simulink model "Model14DOF"  (R2021b)
settings: Solver=ode23tb  StartTime=0.0  StopTime=15  RelTol=1e-3
values from neighbouring files (symbols this model uses):
  InitialLatPosition = 0    [Init_Parameters.m]
  numWheels = 4    [Init_Parameters.m]    (also in VehicleParameters.m)
  TrackWidth = VEH.TrackWidth    [Init_Parameters.m]
  VEH = data.VEH    [Init_Parameters.m]    (also in ModelWorkspace.mat = ; VehicleParameters.m)
  wheelB = VEH.FrontAxlePositionfromCG+VEH.RearAxlePositionfromCG    [Init_Parameters.m]    (also in VehicleParameters.m)
undefined symbols (not defined in the file or in its folder): degtorad
libraries: sharedtransform x5, autolibutils x3, vehdynlibsuspension x2, shared6dof x2, vehdynlibeom x1, vehdynlibtire x1, vehdynlibtirecommon x1
(part 1 of 2)
settings Model: Creator=monic  LastModifiedBy=monic

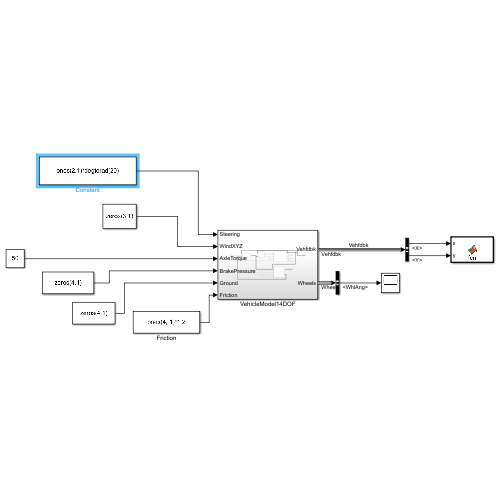
[thumbnail: Simulink's stored preview of the top-level diagram]
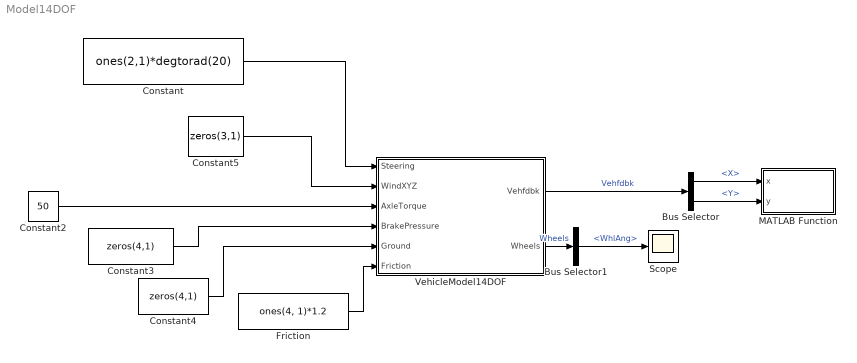
== system Model14DOF ==
  Bus Selector : BusSelector  OutputSignals=InertFrm.Cg.Disp.X,InertFrm.Cg.Disp.Y
  Bus Selector1 : BusSelector  OutputSignals=Steering.WhlAng
  Constant : Constant  Value=ones(2,1)*degtorad(20)
  Constant2 : Constant  Value=50
  Constant3 : Constant  Value=zeros(4,1)
  Constant4 : Constant  Value=zeros(4,1)
  Constant5 : Constant  Value=zeros(3,1)
  Friction : Constant  Value=ones(4, 1)*1.2
  MATLAB Function : MATLAB Function  TreatAsAtomicUnit=on
  Scope : Scope
  VehicleModel14DOF : Subsystem
  wires:
  Constant/1 -> VehicleModel14DOF/1(Steering)
  Constant5/1 -> VehicleModel14DOF/2(WindXYZ)
  Constant2/1 -> VehicleModel14DOF/3(AxleTorque)
  Constant3/1 -> VehicleModel14DOF/4(BrakePressure)
  Constant4/1 -> VehicleModel14DOF/5(Ground)
  Friction/1 -> VehicleModel14DOF/6(Friction)
  VehicleModel14DOF/2(Wheels) -> Bus Selector1/1  "Wheels"
  VehicleModel14DOF/1(Vehfdbk) -> Bus Selector/1  "Vehfdbk"
  Bus Selector/2 -> MATLAB Function/2(y)  "<Y>"
  Bus Selector/1 -> MATLAB Function/1(x)  "<X>"
  Bus Selector1/1 -> Scope/1  "<WhlAng>"

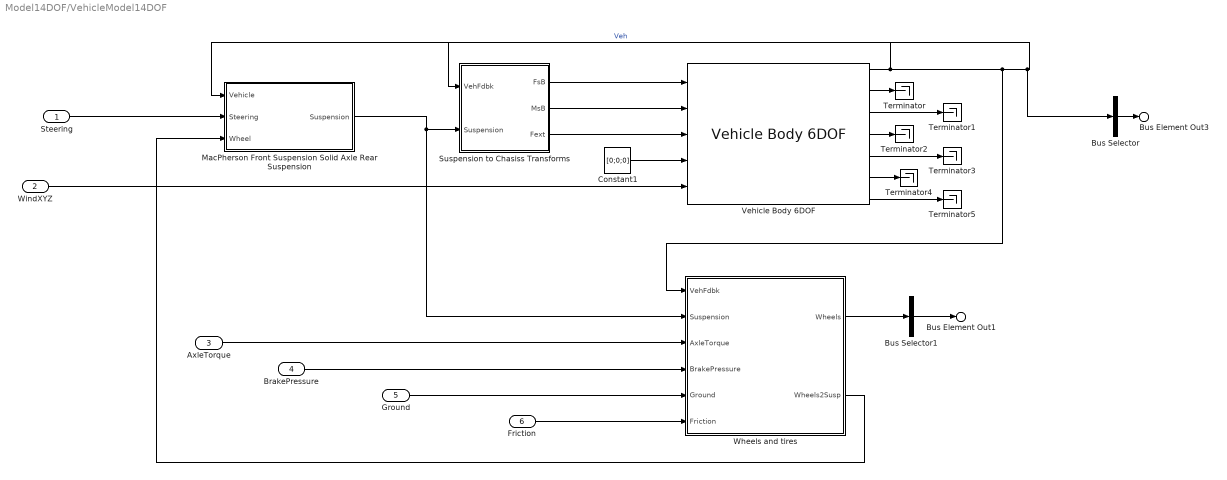
== system Model14DOF/VehicleModel14DOF ==
  Steering : Inport
  WindXYZ : Inport  Port=2
  AxleTorque : Inport  Port=3
  BrakePressure : Inport  Port=4
  Ground : Inport  Port=5
  Friction : Inport  Port=6
  Bus Selector : BusSelector  OutputSignals=InertFrm,BdyFrm  OutputAsBus=on
  Bus Selector1 : BusSelector  OutputSignals=TireFrame,Steering  OutputAsBus=on
  Constant1 : Constant  Value=[0;0;0]
  MacPherson Front Suspension Solid Axle Rear Suspension : Subsystem
  Suspension to Chasiss Transforms : Subsystem
  Terminator{,1..5} (6 alike) : Terminator
  Vehicle Body 6DOF : vehdynlibeom/Vehicle Body 6DOF  extPos=on  extVel=on  extEuler=on  extRotRate=on  htchFMode=off  htchMMode=off  m=VEH.Mass  a=VEH.FrontAxlePositionfromCG  b=VEH.RearAxlePositionfromCG  d=0  h=VEH.HeightCG  dh=1  hl=0  hh=0.1  Xe_o=[VEH.InitialLongPosition,InitialLatPosition,VEH.InitialVertPosition]  xbdot_o=[VEH.InitialLongVel,VEH.InitialLatVel,VEH.InitialVertVel]  eul_o=[VEH.InitialRollAngle,VEH.InitialPitchAngle,VEH.InitialYawAngle]  p_o=[VEH.InitialRollRate,VEH.InitialPitchRate,VEH.InitialYawRate]  Iveh=[VEH.RollMomentInertia 0 0; 0 VEH.PitchMomentInertia 0; 0 0 VEH.YawMomentInertia]  w=VEH.TrackWidth.*[1 1]  z1m=0  z1R=[-.25,.125,.15]  z1I=[1.4,-.2,.1;-.2,1.4,.1;.1,.1,2.25].*0  z2m=0  z2R=[1.4,0,.8]  z2I=[1.4,-.2,.1;-.2,1.4,.1;.1,.1,2.25].*0  z3m=0  z3R=[.75,-.5,.4]  z3I=[5,-.1,-2;-2,9,.1;-.1,.1,6].*0  z4m=0  z4R=[.75,.5,.4]  z4I=[5,-.1,-2;-2,9,.1;-.1,.1,6].*0  z5m=0  z5R=[1.25,-.5,.4]  z5I=[5,-.1,-2;-2,9,.1;-.1,.1,6].*0  z6m=0  z6R=[1.25,-.5,.4]  z6I=[5,-.1,-2;-2,9,.1;-.1,.1,6].*0  z7m=0  z7R=[2,0,.25]  z7I=[1.4,-.2,.1;-.2,1.4,.1;.1,.1,2.25].*0  Af=VEH.FrontalArea  Cd=.3  Cl=.1  Cpm=.1  beta_w=[0 0.01:0.01:0.3]  Cs=[0 0.01:0.01:0.3]  Cym=[0 1e-6:0.01:0.3]  Pabs=101325  extTamb=off  Tair=273  g=9.81  xdot_tol=.1  longOff=0  latOff=0  vertOff=0.0112  wrapAng=off  aMode=2
      settings: SourceProductBaseCode=VE
  Wheels and tires : Subsystem
  Bus Element Out3 : Outport  PortName=Vehfdbk
  Bus Element Out1 : Outport  Port=2  PortName=Wheels
  wires:
  Ground/1 -> Wheels and tires/5(Ground)
  MacPherson Front Suspension Solid Axle Rear Suspension/1(Suspension) -> Wheels and tires/2(Suspension), Suspension to Chasiss Transforms/2(Suspension)
  Vehicle Body 6DOF/3 -> Terminator1/1
  Suspension to Chasiss Transforms/3(Fext) -> Vehicle Body 6DOF/3
  Vehicle Body 6DOF/7 -> Terminator5/1
  BrakePressure/1 -> Wheels and tires/4(BrakePressure)
  AxleTorque/1 -> Wheels and tires/3(AxleTorque)
  Vehicle Body 6DOF/6 -> Terminator4/1
  Vehicle Body 6DOF/5 -> Terminator3/1
  Constant1/1 -> Vehicle Body 6DOF/4
  Wheels and tires/2(Wheels2Susp) -> MacPherson Front Suspension Solid Axle Rear Suspension/3(Wheel)
  Vehicle Body 6DOF/4 -> Terminator2/1
  Suspension to Chasiss Transforms/1(FsB) -> Vehicle Body 6DOF/1
  Vehicle Body 6DOF/2 -> Terminator/1
  Suspension to Chasiss Transforms/2(MsB) -> Vehicle Body 6DOF/2
  WindXYZ/1 -> Vehicle Body 6DOF/5
  Steering/1 -> MacPherson Front Suspension Solid Axle Rear Suspension/2(Steering)
  Friction/1 -> Wheels and tires/6(Friction)
  Wheels and tires/1(Wheels) -> Bus Selector1/1
  Bus Selector1/1 -> Bus Element Out1/1
  Vehicle Body 6DOF/1 -> Wheels and tires/1(VehFdbk), Bus Selector/1, MacPherson Front Suspension Solid Axle Rear Suspension/1(Vehicle), Suspension to Chasiss Transforms/1(VehFdbk)  "Veh"
  Bus Selector/1 -> Bus Element Out3/1

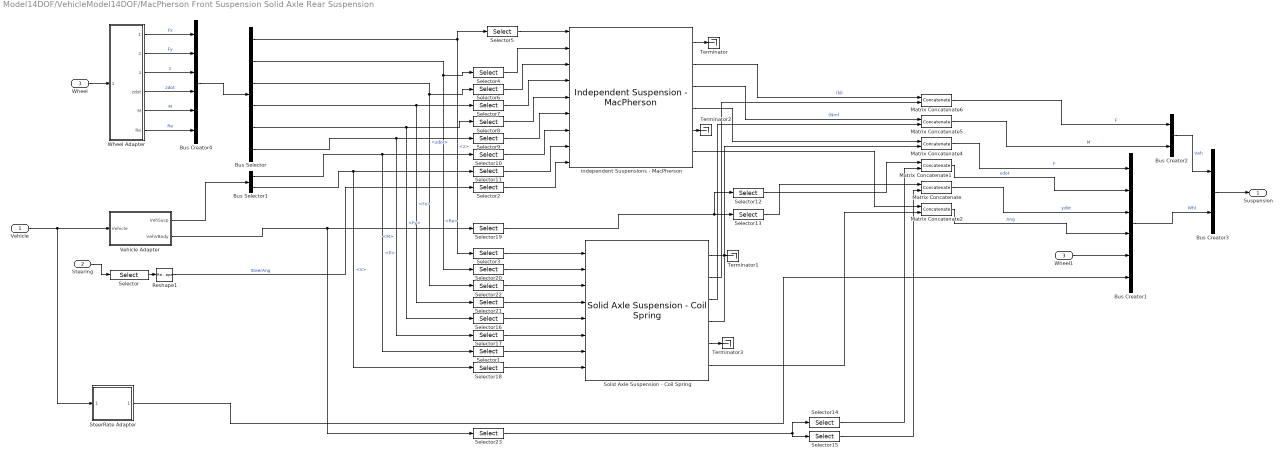
== system Model14DOF/VehicleModel14DOF/MacPherson Front Suspension Solid Axle Rear Suspension ==
  Vehicle : Inport
  Steering : Inport  Port=2
  Wheel : Inport  Port=3
  Bus Creator1 : BusCreator  Inputs=6
  Bus Creator2 : BusCreator  Inputs=2
  Bus Creator3 : BusCreator  Inputs=2
  Bus Creator4 : BusCreator  Inputs=6
  Bus Selector : BusSelector  OutputSignals=z,Re,zdot,Fx,Fy,M
  Bus Selector1 : BusSelector  OutputSignals=P,V
  Matrix Concatenate{,1..2,4..6} (6 alike) : Concatenate  Mode=Multidimensional array  ConcatenateDimension=2
  Reshape1 : Reshape  OutputDimensionality=Row vector (2-D)
  Selector{,2,4..8} (7 alike) : Selector  IndexOptions=Index vector (dialog)  Indices=[1 2]  OutputSizes=1
  Selector{1,17..18,23} (4 alike) : Selector  NumberOfDimensions=2  IndexOptions=Select all,Index vector (dialog)  Indices=[1 2],[3 4]  OutputSizes=1,1
  Selector{9..11,19} (4 alike) : Selector  NumberOfDimensions=2  IndexOptions=Select all,Index vector (dialog)  Indices=[1 2],[1 2]  OutputSizes=1,1
  Selector12 : Selector  NumberOfDimensions=2  InputPortWidth=3  IndexOptions=Index vector (dialog),Select all  Indices=1,1  OutputSizes=1,1
  Selector13 : Selector  NumberOfDimensions=2  InputPortWidth=3  IndexOptions=Index vector (dialog),Select all  Indices=2,1  OutputSizes=1,1
  Selector14 : Selector  NumberOfDimensions=2  InputPortWidth=3  IndexOptions=Index vector (dialog),Select all  Indices=1,1  OutputSizes=1,1
  Selector15 : Selector  NumberOfDimensions=2  InputPortWidth=3  IndexOptions=Index vector (dialog),Select all  Indices=2,1  OutputSizes=1,1
  Selector{3,16,20..22} (5 alike) : Selector  IndexOptions=Index vector (dialog)  Indices=[3 4]  OutputSizes=1
  Solid Axle Suspension - Coil Spring : vehdynlibsuspension/Solid Axle Suspension - Coil Spring  NumAxl=1  NumTracksByAxl=2  StrgEnByAxl=0  TrackNumVec="[1  2]"  AxleNumVec="[1  1]"  SuspTypesByAxle=[1]  SuspImage=suspsacoil.png  AxlIxx=AxlIxx  AxlM=AxlM  TrackCoords=[0 0;VEH.TrackWidth*[-1 1]/2;0 0]  SuspCoords=[0 0;VEH.TrackWidth*[-1 1]/2;0 0]  KzWhlAxl=KzWhlAxl  F0zWhlAxl=F0zWhlAxl  CzWhlAxl=CzWhlAxl  IdealSuspEn=on  IdealSuspAxles=[1]  Kz=Kz  F0z=F0zCS  Cz=Cz  Hmax=Hmax  Toe=0.  RollStrgSlp=0.  ToeStrgSlp=0  Caster=0.  CasterHslp=0.  CasterStrgSlp=0.01  Camber=0.  CamberHslp=0.  CamberStrgSlp=0.01  StrgHgtSlp=0.1432  MappedSuspEn=off  MappedSuspAxles="[1  2]"  f_susp_axl_bp=[1 2]  f_susp_dz_bp=[-0.15 -0.14 -0.13 -0.12 -0.11 -0.10 -0.09 -0.08 -0.07 -0.06 -0.05 -0.04 -0.03 -0.02 -0.01 0.00 0.01 0.02 0.03 0.04 0.05 0.06 0.07 0.08 0.09 0.10 0.11 0.12 0.13 0.14 0.15]  f_susp_dzdot_bp=[-0.15 -0.14 -0.13 -0.12 -0.11 -0.10 -0.09 -0.08 -0.07 -0.06 -0.05 -0.04 -0.03 -0.02 -0.01 0.00 0.01 0.02 0.03 0.04 0.05 0.06 0.07 0.08 0.09 0.10 0.11 0.12 0.13 0.14 0.15]  f_susp_fmz=zeros(31,31,61,2,4)  f_susp_geom=zeros(31,61,2,3)  f_susp_strgdelta_bp=[-30,-29,-28,-27,-26,-25,-24,-23,-22,-21,-20,-19,-18,-17,-16,-15,-14,-13,-12,-11,-10,-9,-8,-7,-6,-5,-4,-3,-2,-1,0,1,2,3,4,5,6,7,8,9,10,11,12,13,14,15,16,17,18,19,20,21,22,23,24,25,26,27,28,29,30]
      settings: SourceProductBaseCode=VE
  SteerRate Adapter : Subsystem
  Terminator{,1..3} (4 alike) : Terminator
  Vehicle Adapter : Subsystem
  Wheel Adapter : Subsystem
  Wheel1 : InportShadow  Port=3
  independent Suspensions - MacPherson : vehdynlibsuspension/Independent Suspension - MacPherson  ActiveDampEn=off  NumAxl=1  NumTracksByAxl=2  StrgEnByAxl=1  AntiSwayEnByAxl=1  TrackNumVec="[1  2]"  AxleNumVec="[1  1]"  SuspTypesByAxle=[1]  SuspImage=suspmacp.png  IdealSuspEn=on  IdealSuspAxles=[1]  Kz=Kz  F0z=F0zMP  Cz=Cz  Hmax=Hmax  f_act_susp_cz=[10000 10000;10000 10000]  f_act_susp_duty_bpt=[0 1]  f_act_susp_zdot_bpt=[-1 1]  Toe=0  RollStrgSlp=0.  ToeStrgSlp=0.  Caster=0.  CasterHslp=0.  CasterStrgSlp=0.  Camber=-0.5*pi/180*0  CamberHslp=0.  CamberStrgSlp=0.  StrgHgtSlp=0.1432  MappedSuspEn=off  MappedSuspAxles="[1  2]"  f_susp_axl_bp=[1 2]  f_susp_dz_bp=[-0.15 -0.14 -0.13 -0.12 -0.11 -0.10 -0.09 -0.08 -0.07 -0.06 -0.05 -0.04 -0.03 -0.02 -0.01 0.00 0.01 0.02 0.03 0.04 0.05 0.06 0.07 0.08 0.09 0.10 0.11 0.12 0.13 0.14 0.15]  f_susp_dzdot_bp=[-0.15 -0.14 -0.13 -0.12 -0.11 -0.10 -0.09 -0.08 -0.07 -0.06 -0.05 -0.04 -0.03 -0.02 -0.01 0.00 0.01 0.02 0.03 0.04 0.05 0.06 0.07 0.08 0.09 0.10 0.11 0.12 0.13 0.14 0.15]  f_susp_fmz=zeros(31,31,61,2,4)  f_susp_geom=zeros(31,61,2,3)  f_susp_strgdelta_bp=[-30,-29,-28,-27,-26,-25,-24,-23,-22,-21,-20,-19,-18,-17,-16,-15,-14,-13,-12,-11,-10,-9,-8,-7,-6,-5,-4,-3,-2,-1,0,1,2,3,4,5,6,7,8,9,10,11,12,13,14,15,16,17,18,19,20,21,22,23,24,25,26,27,28,29,30]  AntiSwayR=0.2  AntiSwayNtrlAng=0.5236  AntiSwayTrsK=8e+02
      settings: SourceProductBaseCode=VE
  Suspension : Outport  VectorParamsAs1DForOutWhenUnconnected=off
  wires:
  Wheel1/1 -> Bus Creator1/5
  Bus Selector/5 -> Selector16/1, Selector8/1  "<Fy>"
  Vehicle Adapter/2(VehVBody) -> Selector23/1, Selector19/1
  Matrix Concatenate1/1 -> Bus Creator1/2  "xdot"
  Selector19/1 -> Selector12/1, Selector13/1
  Selector2/1 -> independent Suspensions - MacPherson/9
  Wheel Adapter/2(WhFy) -> Bus Creator4/2  "Fy"
  Selector11/1 -> independent Suspensions - MacPherson/8
  Bus Creator4/1 -> Bus Selector/1
  Bus Selector/2 -> Selector20/1, Selector4/1  "<Re>"
  Bus Selector1/2 -> Selector18/1, Selector11/1  "<V>"
  Solid Axle Suspension - Coil Spring/3 -> Matrix Concatenate5/2
  Vehicle/1 -> SteerRate Adapter/1(Vehicle), Vehicle Adapter/1(Vehicle)
  Solid Axle Suspension - Coil Spring/6 -> Matrix Concatenate2/2
  Solid Axle Suspension - Coil Spring/1 -> Terminator1/1
  Matrix Concatenate/1 -> Bus Creator1/3  "ydot"
  independent Suspensions - MacPherson/1 -> Terminator/1
  Wheel Adapter/5(M) -> Bus Creator4/5  "M"
  Selector10/1 -> independent Suspensions - MacPherson/7
  Selector23/1 -> Selector15/1, Selector14/1
  Wheel/1 -> Wheel Adapter/1(Wheels)
  Wheel Adapter/4(zdot) -> Bus Creator4/4  "zdot"
  Selector17/1 -> Solid Axle Suspension - Coil Spring/6
  Wheel Adapter/1(WhFx) -> Bus Creator4/1  "Fx"
  Selector20/1 -> Solid Axle Suspension - Coil Spring/2
  Selector6/1 -> independent Suspensions - MacPherson/3
  Selector15/1 -> Matrix Concatenate/2
  Steering/1 -> Selector/1
  Selector18/1 -> Solid Axle Suspension - Coil Spring/8
  Selector16/1 -> Solid Axle Suspension - Coil Spring/5
  Selector7/1 -> independent Suspensions - MacPherson/4
  Matrix Concatenate4/1 -> Bus Creator1/1  "F"
  Solid Axle Suspension - Coil Spring/4 -> Matrix Concatenate4/2
  Selector8/1 -> independent Suspensions - MacPherson/5
  independent Suspensions - MacPherson/2 -> Matrix Concatenate6/1  "(N)"
  Selector5/1 -> independent Suspensions - MacPherson/1
  Selector9/1 -> independent Suspensions - MacPherson/6
  Selector21/1 -> Solid Axle Suspension - Coil Spring/4
  Bus Selector1/1 -> Selector1/1, Selector10/1  "<P>"
  Selector3/1 -> Solid Axle Suspension - Coil Spring/1
  Solid Axle Suspension - Coil Spring/5 -> Terminator3/1
  Selector/1 -> Reshape1/1
  Bus Creator2/1 -> Bus Creator3/1  "Veh"
  Wheel Adapter/3(z) -> Bus Creator4/3  "z"
  Bus Selector/3 -> Selector22/1, Selector6/1  "<zdot>"
  Wheel Adapter/6(Re) -> Bus Creator4/6  "Re"
  Selector22/1 -> Solid Axle Suspension - Coil Spring/3
  Matrix Concatenate5/1 -> Bus Creator2/2  "M"
  independent Suspensions - MacPherson/4 -> Matrix Concatenate4/1
  Selector4/1 -> independent Suspensions - MacPherson/2
  Selector1/1 -> Solid Axle Suspension - Coil Spring/7
  Bus Selector/1 -> Selector3/1, Selector5/1  "<z>"
  Bus Selector/6 -> Selector17/1, Selector9/1  "<M>"
  Matrix Concatenate6/1 -> Bus Creator2/1  "F"
  Bus Creator3/1 -> Suspension/1
  Bus Selector/4 -> Selector21/1, Selector7/1  "<Fx>"
  Reshape1/1 -> Selector2/1  "SteerAng"
  independent Suspensions - MacPherson/5 -> Terminator2/1
  Vehicle Adapter/1(VehSusp) -> Bus Selector1/1
  Bus Creator1/1 -> Bus Creator3/2  "Whl"
  independent Suspensions - MacPherson/3 -> Matrix Concatenate5/1  "(Nm)"
  Selector12/1 -> Matrix Concatenate1/1
  Matrix Concatenate2/1 -> Bus Creator1/4  "Ang"
  Solid Axle Suspension - Coil Spring/2 -> Matrix Concatenate6/2
  Selector14/1 -> Matrix Concatenate1/2
  independent Suspensions - MacPherson/6 -> Matrix Concatenate2/1
  Selector13/1 -> Matrix Concatenate/1
  SteerRate Adapter/1(AngVel) -> Bus Creator1/6

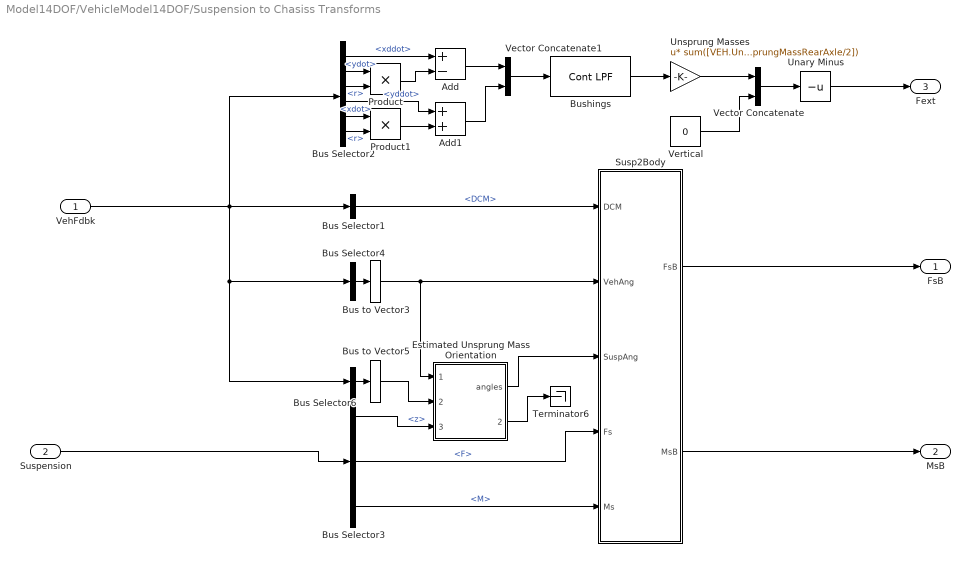
== system Model14DOF/VehicleModel14DOF/Suspension to Chasiss Transforms ==
  VehFdbk : Inport
  Suspension : Inport  Port=2
  Add : Sum  Inputs=+-
  Add1 : Sum
  Bus Selector1 : BusSelector  OutputSignals=BdyFrm.Cg.DCM
  Bus Selector2 : BusSelector  OutputSignals=BdyFrm.Cg.Acc.xddot,BdyFrm.Cg.Vel.ydot,BdyFrm.Cg.AngVel.r,BdyFrm.Cg.Acc.yddot,BdyFrm.Cg.Vel.xdot,BdyFrm.Cg.AngVel.r
  Bus Selector3 : BusSelector  OutputSignals=Whl.signal5.SuspFrame.z,Veh.F,Veh.M
  Bus Selector4 : BusSelector  OutputSignals=InertFrm.Cg.Ang.phi,InertFrm.Cg.Ang.theta,InertFrm.Cg.Ang.psi  OutputAsBus=on
  Bus Selector6 : BusSelector  OutputSignals=InertFrm.Geom.Disp.X,InertFrm.Geom.Disp.Y,InertFrm.Geom.Disp.Z  OutputAsBus=on
  Bus to Vector3 : BusToVector
  Bus to Vector5 : BusToVector
  Bushings : autolibutils/Cont LPF  wc=40*pi  aMode=2
      settings: SourceProductBaseCode=PW,DR,MT,UV,VE
  Estimated Unsprung Mass Orientation : MATLAB Function  TreatAsAtomicUnit=on
  Product : Product
  Product1 : Product
  Susp2Body : Subsystem
  Terminator6 : Terminator
  Unary Minus : UnaryMinus
  Unsprung Masses : Gain  Gain=sum([VEH.UnsprungMassFrontAxle/2 VEH.UnsprungMassFrontAxle/2 VEH.UnsprungMassRearAxle/2 VEH.UnsprungMassRearAxle/2])  Multiplication=Matrix(u*K)
  Vector Concatenate : Concatenate
  Vector Concatenate1 : Concatenate
  Vertical : Constant  Value=0
  FsB : Outport
  MsB : Outport  Port=2
  Fext : Outport  Port=3
  wires:
  Estimated Unsprung Mass Orientation/1(angles) -> Susp2Body/3(SuspAng)
  Bus Selector3/1 -> Estimated Unsprung Mass Orientation/3(Ground)  "<z>"
  Vector Concatenate1/1 -> Bushings/1
  Bus Selector2/6 -> Product1/2  "<r>"
  Product/1 -> Add/2
  Bus Selector2/3 -> Product/2  "<r>"
  Bus Selector2/5 -> Product1/1  "<xdot>"
  Vertical/1 -> Vector Concatenate/2
  Add1/1 -> Vector Concatenate1/2
  Suspension/1 -> Bus Selector3/1
  Bushings/1 -> Unsprung Masses/1
  Vector Concatenate/1 -> Unary Minus/1
  VehFdbk/1 -> Bus Selector6/1, Bus Selector4/1, Bus Selector2/1, Bus Selector1/1
  Product1/1 -> Add1/2
  Bus to Vector3/1 -> Estimated Unsprung Mass Orientation/1(angleIn), Susp2Body/2(VehAng)
  Bus to Vector5/1 -> Estimated Unsprung Mass Orientation/2(GemoXYZIn)
  Unary Minus/1 -> Fext/1
  Bus Selector2/1 -> Add/1  "<xddot>"
  Add/1 -> Vector Concatenate1/1
  Bus Selector3/3 -> Susp2Body/5(Ms)  "<M>"
  Bus Selector2/2 -> Product/1  "<ydot>"
  Unsprung Masses/1 -> Vector Concatenate/1
  Estimated Unsprung Mass Orientation/2(GeomXYZ) -> Terminator6/1
  Bus Selector2/4 -> Add1/1  "<yddot>"
  Bus Selector3/2 -> Susp2Body/4(Fs)  "<F>"
  Bus Selector1/1 -> Susp2Body/1(DCM)  "<DCM>"
  Bus Selector6/1 -> Bus to Vector5/1
  Bus Selector4/1 -> Bus to Vector3/1
  Susp2Body/1(FsB) -> FsB/1
  Susp2Body/2(MsB) -> MsB/1

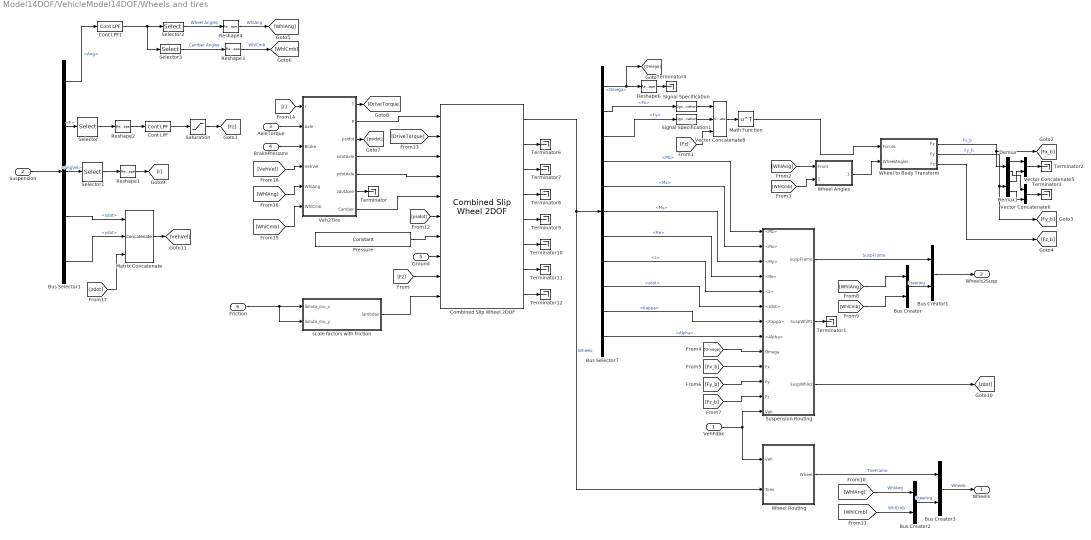
== system Model14DOF/VehicleModel14DOF/Wheels and tires ==
  VehFdbk : Inport
  Suspension : Inport  Port=2
  AxleTorque : Inport  Port=3
  BrakePressure : Inport  Port=4
  Ground : Inport  Port=5
  Friction : Inport  Port=6
  Bus Creator{,1..3} (4 alike) : BusCreator  Inputs=2
  Bus Selector1 : BusSelector  OutputSignals=Whl.Ang,Whl.F,Whl.AngVel,Whl.xdot,Whl.ydot
  Bus Selector7 : BusSelector  OutputSignals=Omega,Fx,Fy,Mz,Mx,My,Re,z,zdot,Kappa,Alpha
  Combined Slip Wheel 2DOF : vehdynlibtire/Combined Slip Wheel 2DOF  tireType=Light passenger car 205/60R15  BrakeType=Disc  plySteer=off  turnslip=off  mu_static=.3  mu_kinetic=.2  disk_abore=.05  Rm=.177  num_pads=2  drum_abore=0.0508  drum_a=0.123  drum_c=0.212  drum_r=0.15  drum_theta1=0  drum_theta2=126  brake_p_bpt=[1 11.4736842105263 21.9473684210526 32.4210526315789 42.8947368421053 53.3684210526316 63.8421052631579 74.3157894736842 84.7894736842105 95.2631578947368 105.736842105263 116.210526315789 126.684210526316 137.157894736842 147.631578947368 158.105263157895 168.578947368421 179.052631578947 189.526315789474 200]  brake_n_bpt=[0 52.6315789473684 105.263157894737 157.894736842105 210.526315789474 263.157894736842 315.789473684211 368.421052631579 421.052631578947 473.684210526316 526.315789473684 578.947368421053 631.578947368421 684.210526315789 736.842105263158 789.473684210526 842.105263157895 894.736842105263 947.368421052632 1000]  f_brake_t=[43.4900602404453 42.5056030554862 41.5350898940194 40.5780454442085 39.6340111501808 38.7025443887544 37.7832176914519 36.8756180088306 35.9793460143796 35.0940154454303 34.2192524787115 33.3546951383474 32.4999927342521 31.6548053290159 30.8188032315107 29.991666515561 29.1730845621415 28.362755623661 27.5603864089927 26.765691687993;498.991217495636 487.695866636631 476.560505099801 465.579679307235 454.748127933653 444.060772460445 433.51270824929 423.099196101319 412.81565427025 402.657650900201 392.620896861006 382.701238955775 372.894653477208 363.197240090814 353.605216024701 344.114910546964 334.722759712992 325.425301366216 316.219170376863 307.10109410434;954.492374750826 932.886130217776 911.585920305583 890.581313170261 869.862244717126 849.419000532136 829.242198807128 809.322774193808 789.651962526121 770.221286354971 751.0225412433 732.047782773203 713.289314220164 694.739674852612 676.391628817892 658.238154578366 640.272434863842 622.48784710877 604.877954344734 587.436496520688;1409.99353200602 1378.07639379892 1346.61133551136 1315.58294703329 1284.9763615006 1254.77722860383 1224.97168936497 1195.5463522863 1166.48827078199 1137.78492180974 1109.42418562559 1081.39432659063 1053.68397496312 1026.28210961441 999.178041611083 972.361398609768 945.822110014692 919.550392851325 893.536738312604 867.771898937035;1865.49468926121 1823.26665738007 1781.63675071715 1740.58458089631 1700.09047828407 1660.13545667552 1620.7011799228 1581.76993037878 1543.32457903786 1505.34855726451 1467.82583000789 1430.74087040806 1394.07863570608 1357.82454437621 1321.96445440427 1286.48464264117 1251.37178516554 1216.61293859388 1182.19552228048 1148.10730135338;2320.9958465164 2268.45692096121 2216.66216592293 2165.58621475934 2115.20459506754 2065.49368474721 2016.43067048064 1967.99350847127 1920.16088729373 1872.91219271928 1826.22747439018 1780.08741422549 1734.47329644903 1689.36697913801 1644.75086719747 1600.60788667257 1556.92146031639 1513.67548433643 1470.85430624835 1428.44270376973;2776.49700377159 2713.64718454235 2651.68758112871 2590.58784862237 2530.31871185102 2470.8519128189 2412.16016103848 2354.21708656376 2296.9971955496 2240.47582817405 2184.62911877248 2129.43395804292 2074.86795719199 2020.9094138998 1967.53727999066 1914.73113070398 1862.47113546724 1810.73803007899 1759.51309021622 1708.77810618608;3231.99816102678 3158.8374481235 3086.71299633449 3015.58948248539 2945.43282863449 2876.21014089059 2807.88965159632 2740.44066465625 2673.83350380547 2608.03946362882 2543.03076315477 2478.78050186034 2415.26261793494 2352.4518486616 2290.32369278385 2228.85437473538 2168.02081061809 2107.80057582154 2048.17187418409 1989.11350860242;3687.49931828197 3604.02771170464 3521.73841154027 3440.59111634842 3360.54694541796 3281.56836896228 3203.61914215416 3126.66424274874 3050.66981206134 2975.60309908359 2901.43240753707 2828.12704567777 2755.6572786779 2683.9942834234 2613.11010557704 2542.97761876678 2473.57048576894 2404.8631215641 2336.83065815196 2269.44891101877;4143.00047553716 4049.21797528579 3956.76382674606 3865.59275021144 3775.66106220143 3686.92659703397 3599.34863271199 3512.88782084123 3427.50612031721 3343.16673453836 3259.83405191936 3177.4735894952 3096.05193942085 3015.5367181852 2935.89651837023 2857.10086279818 2779.12016091979 2701.92566730665 2625.48944211983 2549.78431343512;4598.50163279235 4494.40823886693 4391.78924195184 4290.59438407447 4190.77517898491 4092.28482510566 3995.07812326983 3899.11139893372 3804.34242857308 3710.73036999313 3618.23569630166 3526.82013331263 3436.44660016381 3347.079152947 3258.68293116342 3171.22410682959 3084.66983607064 2998.98821304921 2914.1482260877 2830.11971585147;5054.00279004754 4939.59850244808 4826.81465715762 4715.59601793749 4605.88929576838 4497.64305317735 4390.80761382767 4285.3349770262 4181.17873682896 4078.2940054479 3976.63734068395 3876.16667713006 3776.84126090677 3678.62158770879 3581.46934395661 3485.34735086099 ...(+2764 chars)]  tireParamSet=vdynPassCar.mat  PRESMAX=1000000  PRESMIN=10000  FZMAX=10000  FZMIN=100  VXLOW=.1  KPUMAX=1.5  KPUMIN=-1.5  ALPMAX=1.5  ALPMIN=-1.5  CAMMAX=0.2  CAMMIN=-0.2  LONGVL=16.7  FxRelFreqLwrLim=200*pi  FyRelFreqLwrLim=50*pi  MyRelFreqLwrLim=100*pi  omegao=0  br=1e-3  UNLOADED_RADIUS=0.30938  NOMPRES=220000  FNOMIN=4000  WIDTH=0.20905  RIM_RADIUS=0.1914  MASS=9.4649  IYY=0.74063  GRAVITY=-9.81  zo=.015+VEH.InitialVertPosition  zdoto=0  BREFF=8.25094594147963  DREFF=0.260468730454265  FREFF=0.0735298544471851  Q_RE0=1.00866439868088  Q_V1=0.000760413786224011  Q_V2=0.0463384792019201  Q_FZ1=0  Q_FZ2=15.6870832810226  Q_FZ3=0  Q_FCX=0.138643970247602  Q_FCY=0.10843499565426  Q_FCY2=-0.465763352339538  PFZ1=0.69958166705601  VERTICAL_STIFFNESS=207885.061134007  VERTICAL_DAMPING=500  BOTTOM_OFFST=0.00990653336182505  BOTTOM_STIFF=1999075.87051971  LONGITUDINAL_STIFFNESS=388714.175879854  LATERAL_STIFFNESS=157087.404633332  PCFX1=0.18539229191199  PCFX2=0  PCFX3=0  PCFY1=0.163183345037677  PCFY2=0  PCFY3=0.249094918231954  Q_RA1=0.675942571700787  Q_RA2=0.73800463546164  Q_RB1=1.04487486456705  Q_RB2=-1.191763806629  PCX1=1.58523057950359  PDX1=1.0239116238178  PDX2=-0.0842405110022724  PDX3=0  PEX1=0.110312777158455  PEX2=0.313468516038146  PEX3=0  PEX4=0.0016060905760045  PKX1=21.3872544684023  PKX2=14.0006541873175  PKX3=-0.405326109653452  PHX1=0.000212599305364818  PHX2=0.00115950515263055  PVX1=1.59236164471432e-05  PVX2=0.000104321112127671  PPX1=-0.349461321276586  PPX2=0.387840040616429  PPX3=-0.0969947336569324  PPX4=0.0632271859795801  RBX1=12.7633329850276  RBX2=9.5787123658471  RBX3=0  RCX1=1.02796280922059  REX1=-0.45202516851367  REX2=-0.47304886171176  RHX1=0.000233272373115809  QSX1=-0.00788307788961443  QSX2=0.954629515459396  QSX3=0.0155855777667025  QSX4=0.125904607142414  QSX5=1.01110069703963  QSX6=20.1938577118433  QSX7=0.310818120717083  QSX8=-0.0430823751139655  QSX9=0.636494404888216  QSX10=0.142438060591663  QSX11=0.346766530036373  QSX12=0  QSX13=0  QSX14=0  PPMX1=0  PCY1=1.34299950037631  PDY1=0.878267729082195  PDY2=-0.0644597923147385  PDY3=0  PEY1=-0.809776534470972  PEY2=-0.600180598867198  PEY3=0.0991732552633487  PEY4=-6.5577974035573  PEY5=0  PKY1=-15.5714726518315  PKY2=1.73126522291751  PKY3=0.365349873517229  PKY4=1.98176755955416  PKY5=0  PKY6=-0.884005199550313  PKY7=-0.237259727611847  PHY1=-0.00183370557235628  PHY2=0.00346401302716671  PVY1=-0.00675427560163264  PVY2=0.036379218103843  PVY3=-0.163543984089166  PVY4=-0.491003349625726  PPY1=-0.62059646553185  PPY2=-0.0647824842338686  PPY3=-0.164648843290686  PPY4=0.283193909060098  PPY5=0  RBY1=10.7588809173639  RBY2=7.70420065295029  RBY3=3.40283755070691e-06  RBY4=0  RCY1=1.06691874059059  REY1=0.308244924574305  REY2=7.48775032604508e-06  RHY1=0.0118479204960415  RHY2=7.63650177161071e-06  RVY1=0.0560024425050078  RVY2=7.48487127056197e-06  RVY3=0  RVY4=98.4047026517149  RVY5=2.02759273900054  RVY6=15.7623064923347  QSY1=0.00699077564863536  QSY2=0  QSY3=0.00153535478298811  QSY4=8.55710322455322e-05  QSY5=0  QSY6=0  QSY7=0.89443879773793  QSY8=-0.403227641260894  QBZ1=11.666656027484  QBZ2=-1.30355438574485  QBZ3=0  QBZ4=0.177918305399071  QBZ5=-0.162481135068033  QBZ6=0  QBZ9=30.1445534682089  QBZ10=0  QCZ1=1.29026978207574  QDZ1=0.0886972644991399  QDZ2=-0.0058634820161856  QDZ3=0.3805597481383  QDZ4=0  QDZ6=0.00160914918118959  QDZ7=-0.00211036330862154  QDZ8=-0.13921904912557  QDZ9=0.00816585550028243  QDZ10=0  QDZ11=0  QEZ1=-2.19802254534746  QEZ2=1.01850535789165  QEZ3=0  QEZ4=0.278379679112054  QEZ5=-0.548414722765386  QHZ1=0.00148361198869669  QHZ2=0.00202017567585904  QHZ3=0.240316641332066  QHZ4=-0.210114035738085  PPZ1=-0.443927982388615  PPZ2=0  SSZ1=0.00914999585397887  SSZ2=0.0389830656052735  SSZ3=0  SSZ4=0  PDXP1=0.396718274678791  PDXP2=0  PDXP3=0  PKYP1=1.00587060633573  PDYP1=0.40483048923438  PDYP2=0  PDYP3=0  PDYP4=0  PHYP1=0.992731942067188  PHYP2=0.150352945499914  PHYP3=0  PHYP4=-3.98988682633674  PECP1=0.502379254513503  PECP2=0  QDTP1=10.0178654287947  QCRP1=0.200627747200702  QCRP2=0.0995735881599772  QBRP1=0.0997107127960717  QDRP1=1.01432910167423  QDRP2=0  aMode=2
      settings: SourceProductBaseCode=VE
  Cont LPF : autolibutils/Cont LPF  wc=100*2*pi  aMode=2
      settings: SourceProductBaseCode=PW,DR,MT,UV,VE
  Cont LPF1 : autolibutils/Cont LPF  wc=100*2*pi  aMode=2
      settings: SourceProductBaseCode=PW,DR,MT,UV,VE
  Demux : Demux  Outputs=[2,2]
  Demux1 : Demux  Outputs=[2,2]
  Math Function : Math  Operator=transpose  SignedPower=on  SaturateOnIntegerOverflow=on
  Matrix Concatenate : Concatenate  NumInputs=3  Mode=Multidimensional array
  Pressure : vehdynlibtirecommon/Constant  const=220000  numWheels=4
      settings: SourceProductBaseCode=VE
  Reshape{1..4} (4 alike) : Reshape
  Reshape6 : Reshape  OutputDimensionality=Customize  OutputDimensions=[2,2]
  Saturation : Saturate  UpperLimit=inf  LowerLimit=-10*9.81*2000  ZeroCross=off
  Selector : Selector  NumberOfDimensions=2  InputPortWidth=3  IndexOptions=Index vector (dialog),Select all  Indices=[3],1  OutputSizes=1,1
  Selector1 : Selector  NumberOfDimensions=2  InputPortWidth=1  IndexOptions=Index vector (dialog),Select all  Indices=[3],1  OutputSizes=1,1
  Selector2 : Selector  NumberOfDimensions=2  InputPortWidth=3  IndexOptions=Index vector (dialog),Select all  Indices=3,1  OutputSizes=1,1
  Selector3 : Selector  NumberOfDimensions=2  InputPortWidth=3  IndexOptions=Index vector (dialog),Select all  Indices=1,1  OutputSizes=1,1
  Signal Specification : SignalSpecification  Dimensions=4
  Signal Specification1 : SignalSpecification  Dimensions=4
  Suspension Routing : Subsystem
  Terminator{,1..4,6..12} (12 alike) : Terminator
  Vector Concatenate5 : Concatenate  Mode=Multidimensional array  ConcatenateDimension=2
  Vector Concatenate6 : Concatenate  Mode=Multidimensional array  ConcatenateDimension=2
  Vector Concatenate8 : Concatenate  NumInputs=3  Mode=Multidimensional array  ConcatenateDimension=2
  Veh2Tire : Subsystem
  Wheel Angles : Subsystem
  Wheel Routing : Subsystem
  Wheel to Body Transform : Subsystem
  scale factors with friction : Subsystem
  Wheels : Outport  VectorParamsAs1DForOutWhenUnconnected=off
  Wheels2Susp : Outport  Port=2  VectorParamsAs1DForOutWhenUnconnected=off
  wires:
  Combined Slip Wheel 2DOF/6 -> Terminator10/1
  Bus Selector7/1 -> [Omega], Reshape6/1  "<Omega>"
  Combined Slip Wheel 2DOF/3 -> Terminator7/1
  Reshape2/1 -> Cont LPF/1
  Wheel to Body Transform/1(Fx) -> Demux/1, [Fx_b]  "Fx_b"
  Math Function/1 -> Wheel to Body Transform/1(Forces)
  Bus Selector1/2 -> Selector/1  "<F>"
  Cont LPF/1 -> Saturation/1
  Saturation/1 -> [Fz]
  [DriveTorque] -> Combined Slip Wheel 2DOF/2
  Demux/2 -> Vector Concatenate6/1
  Combined Slip Wheel 2DOF/1 -> Wheel Routing/2(Tires), Bus Selector7/1  "Wheels"
  Vector Concatenate6/1 -> Terminator3/1
  Veh2Tire/2(P) -> Combined Slip Wheel 2DOF/1
  Wheel to Body Transform/3(Fz) -> [Fz_b]
  [psidot] -> Combined Slip Wheel 2DOF/6
  [Fz] -> Vector Concatenate8/3
  Combined Slip Wheel 2DOF/5 -> Terminator9/1
  Reshape6/1 -> Terminator4/1
  Combined Slip Wheel 2DOF/7 -> Terminator11/1
  Selector/1 -> Reshape2/1
  Signal Specification/1 -> Vector Concatenate8/1
  Vector Concatenate5/1 -> Terminator2/1
  Demux1/2 -> Vector Concatenate6/2
  Veh2Tire/5(ydotAxle) -> Combined Slip Wheel 2DOF/4
  Pressure/1 -> Combined Slip Wheel 2DOF/7
  Bus Selector7/3 -> Signal Specification1/1  "<Fy>"
  Wheel to Body Transform/2(Fy) -> [Fy_b], Demux1/1  "Fy_b"
  Demux1/1 -> Vector Concatenate5/2
  Vector Concatenate8/1 -> Math Function/1
  Combined Slip Wheel 2DOF/4 -> Terminator8/1
  Demux/1 -> Vector Concatenate5/1
  Veh2Tire/7(Camber) -> Combined Slip Wheel 2DOF/5
  Ground/1 -> Combined Slip Wheel 2DOF/8
  Combined Slip Wheel 2DOF/8 -> Terminator12/1
  Combined Slip Wheel 2DOF/2 -> Terminator6/1
  Signal Specification1/1 -> Vector Concatenate8/2
  Bus Selector7/2 -> Signal Specification/1  "<Fx>"
  [Fz] -> Combined Slip Wheel 2DOF/9
  Wheel Angles/1(Vehicle) -> Wheel to Body Transform/2(WheelAngles)
  Veh2Tire/4(xdotAxle) -> Combined Slip Wheel 2DOF/3
  scale factors with friction/1(lambdas) -> Combined Slip Wheel 2DOF/10
  Suspension/1 -> Bus Selector1/1
  Cont LPF1/1 -> Selector3/1, Selector2/1
  Selector2/1 -> Reshape4/1  "Wheel Angles"
  Reshape3/1 -> [WhlCmb]  "WhlCmb"
  Reshape4/1 -> [WhlAng]  "WhlAng"
  Selector3/1 -> Reshape3/1  "Camber Angles"
  Bus Selector1/1 -> Cont LPF1/1  "<Ang>"
  [WhlAng] -> Wheel Angles/1(Front)
  [WhlCmb] -> Wheel Angles/2(Camber)
  Bus Selector7/4 -> Suspension Routing/1(<Mz>)  "<Mz>"
  Bus Selector7/5 -> Suspension Routing/2(<Mx>)  "<Mx>"
  Bus Selector7/6 -> Suspension Routing/3(<My>)  "<My>"
  Bus Selector7/7 -> Suspension Routing/4(<Re>)  "<Re>"
  Bus Selector7/8 -> Suspension Routing/5(<z>)  "<z>"
  Bus Selector7/9 -> Suspension Routing/6(<zdot>)  "<zdot>"
  Bus Selector7/10 -> Suspension Routing/7(<Kappa>)  "<Kappa>"
  Bus Selector7/11 -> Suspension Routing/8(<Alpha>)  "<Alpha>"
  [Omega] -> Suspension Routing/9(Omega)
  [Fx_b] -> Suspension Routing/10(Fx)
  [Fy_b] -> Suspension Routing/11(Fy)
  [Fz_b] -> Suspension Routing/12(Fz)
  VehFdbk/1 -> Wheel Routing/1(Veh), Suspension Routing/13(Veh)
  Bus Creator1/1 -> Wheels2Susp/1
  Bus Creator/1 -> Bus Creator1/2  "Steering"
  Suspension Routing/1(SuspFrame) -> Bus Creator1/1  "SuspFrame"
  [WhlAng] -> Bus Creator/1
  [WhlCmb] -> Bus Creator/2
  Suspension Routing/2(SuspWhlPz) -> Terminator1/1
  Suspension Routing/3(SuspWhlVz) -> [zdot]
  Bus Creator3/1 -> Wheels/1  "Wheels"
  [WhlAng] -> Bus Creator2/1  "WhlAng"
  Wheel Routing/1(Wheel) -> Bus Creator3/1  "TireFrame"
  Bus Creator2/1 -> Bus Creator3/2  "Steering"
  [WhlCmb] -> Bus Creator2/2  "WhlCmb"
  Veh2Tire/6(zdotAxle) -> Terminator/1
  Veh2Tire/3(psidot) -> [psidot]
  Veh2Tire/1(T) -> [DriveTorque]
  Selector1/1 -> Reshape1/1
  Reshape1/1 -> [r]
  Bus Selector1/3 -> Selector1/1  "<AngVel>"
  [r] -> Veh2Tire/1(r)
  AxleTorque/1 -> Veh2Tire/2(Axle)
  BrakePressure/1 -> Veh2Tire/3(Brake)
  [WhlCmb] -> Veh2Tire/6(WhlCmb)
  [WhlAng] -> Veh2Tire/5(WhlAng)
  Bus Selector1/4 -> Matrix Concatenate/1  "<xdot>"
  Bus Selector1/5 -> Matrix Concatenate/2  "<ydot>"
  [zdot] -> Matrix Concatenate/3
  Matrix Concatenate/1 -> [VehVel]
  [VehVel] -> Veh2Tire/4(VehVel)
  Friction/1 -> scale factors with friction/2(lamda_mu_y), scale factors with friction/1(lamda_mu_x)

== system Model14DOF/VehicleModel14DOF/MacPherson Front Suspension Solid Axle Rear Suspension/SteerRate Adapter ==
  Vehicle : Inport
  Add : Sum
  Bus Selector3 : BusSelector  OutputSignals=BdyFrm.Cg.AngVel.r
  Constant : Constant  Value=zeros(1,4)
  Matrix Concatenate : Concatenate  NumInputs=3  Mode=Multidimensional array
  Matrix Concatenate1 : Concatenate  NumInputs=3  Mode=Multidimensional array
  Reshape2 : Reshape  OutputDimensionality=Row vector (2-D)
  Reshape3 : Reshape  OutputDimensionality=Row vector (2-D)
  Reshape4 : Reshape  OutputDimensionality=Row vector (2-D)
  Selector12 : Selector  InputPortWidth=1  IndexOptions=Index vector (dialog)  Indices=[1 1 1 1]  OutputSizes=1
  SteerRates : Constant  Value=zeros(1,4)
  AngVel : Outport
  wires:
  Reshape2/1 -> Matrix Concatenate1/1, Matrix Concatenate1/3, Matrix Concatenate1/2
  Vehicle/1 -> Bus Selector3/1
  Selector12/1 -> Reshape4/1
  Reshape4/1 -> Matrix Concatenate/3
  Add/1 -> AngVel/1  "AngVel"
  Matrix Concatenate1/1 -> Add/1
  SteerRates/1 -> Reshape2/1
  Reshape3/1 -> Matrix Concatenate/2, Matrix Concatenate/1
  Constant/1 -> Reshape3/1
  Bus Selector3/1 -> Selector12/1  "<r>"
  Matrix Concatenate/1 -> Add/2

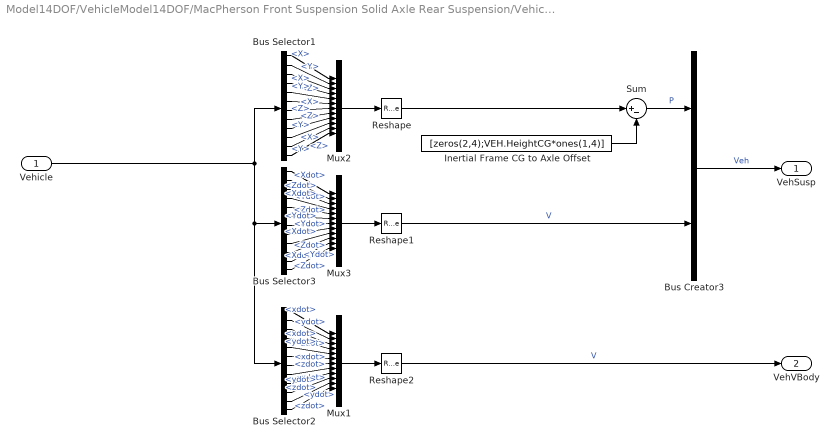
== system Model14DOF/VehicleModel14DOF/MacPherson Front Suspension Solid Axle Rear Suspension/Vehicle Adapter ==
  Vehicle : Inport
  Bus Creator3 : BusCreator  Inputs=2
  Bus Selector1 : BusSelector  OutputSignals=InertFrm.FrntAxl.Lft.Disp.X,InertFrm.FrntAxl.Lft.Disp.Y,InertFrm.FrntAxl.Lft.Disp.Z,InertFrm.FrntAxl.Rght.Disp.X,InertFrm.FrntAxl.Rght.Disp.Y,InertFrm.FrntAxl.Rght.Disp.Z,InertFrm.RearAxl.Lft.Disp.X,InertFrm.RearAxl.Lft.Disp.Y,InertFrm.RearAxl.Lft.Disp.Z,InertFrm.RearAxl.Rght.Disp.X,InertFrm.RearAxl.Rght.Disp.Y,InertFrm.RearAxl.Rght.Disp.Z
  Bus Selector2 : BusSelector  OutputSignals=BdyFrm.FrntAxl.Lft.Vel.xdot,BdyFrm.FrntAxl.Lft.Vel.ydot,BdyFrm.FrntAxl.Lft.Vel.zdot,BdyFrm.FrntAxl.Rght.Vel.xdot,BdyFrm.FrntAxl.Rght.Vel.ydot,BdyFrm.FrntAxl.Rght.Vel.zdot,BdyFrm.RearAxl.Lft.Vel.xdot,BdyFrm.RearAxl.Lft.Vel.ydot,BdyFrm.RearAxl.Lft.Vel.zdot,BdyFrm.RearAxl.Rght.Vel.xdot,BdyFrm.RearAxl.Rght.Vel.ydot,BdyFrm.RearAxl.Rght.Vel.zdot
  Bus Selector3 : BusSelector  OutputSignals=InertFrm.FrntAxl.Lft.Vel.Xdot,InertFrm.FrntAxl.Lft.Vel.Ydot,InertFrm.FrntAxl.Lft.Vel.Zdot,InertFrm.FrntAxl.Rght.Vel.Xdot,InertFrm.FrntAxl.Rght.Vel.Ydot,InertFrm.FrntAxl.Rght.Vel.Zdot,InertFrm.RearAxl.Lft.Vel.Xdot,InertFrm.RearAxl.Lft.Vel.Ydot,InertFrm.RearAxl.Lft.Vel.Zdot,InertFrm.RearAxl.Rght.Vel.Xdot,InertFrm.RearAxl.Rght.Vel.Ydot,InertFrm.RearAxl.Rght.Vel.Zdot
  Inertial Frame CG to Axle Offset : Constant  Value=[zeros(2,4);VEH.HeightCG*ones(1,4)]
  Mux1 : Mux  Inputs=12
  Mux2 : Mux  Inputs=12
  Mux3 : Mux  Inputs=12
  Reshape : Reshape  OutputDimensionality=Customize  OutputDimensions=[3,4]
  Reshape1 : Reshape  OutputDimensionality=Customize  OutputDimensions=[3,4]
  Reshape2 : Reshape  OutputDimensionality=Customize  OutputDimensions=[3,4]
  Sum : Sum  Inputs=|+-
  VehSusp : Outport
  VehVBody : Outport  Port=2
  wires:
  Bus Selector3/8 -> Mux3/8  "<Ydot>"
  Bus Selector3/1 -> Mux3/1  "<Xdot>"
  Bus Selector3/6 -> Mux3/6  "<Zdot>"
  Bus Selector1/1 -> Mux2/1  "<X>"
  Bus Selector1/7 -> Mux2/7  "<X>"
  Bus Selector3/9 -> Mux3/9  "<Zdot>"
  Bus Selector3/2 -> Mux3/2  "<Ydot>"
  Bus Selector1/3 -> Mux2/3  "<Z>"
  Bus Selector2/7 -> Mux1/7  "<xdot>"
  Bus Selector3/7 -> Mux3/7  "<Xdot>"
  Bus Selector3/12 -> Mux3/12  "<Zdot>"
  Vehicle/1 -> Bus Selector3/1, Bus Selector2/1, Bus Selector1/1
  Bus Selector1/2 -> Mux2/2  "<Y>"
  Bus Selector2/3 -> Mux1/3  "<zdot>"
  Bus Selector3/3 -> Mux3/3  "<Zdot>"
  Bus Selector2/5 -> Mux1/5  "<ydot>"
  Bus Selector1/9 -> Mux2/9  "<Z>"
  Reshape2/1 -> VehVBody/1  "V"
  Bus Selector2/6 -> Mux1/6  "<zdot>"
  Bus Selector1/5 -> Mux2/5  "<Y>"
  Inertial Frame CG to Axle Offset/1 -> Sum/2
  Bus Selector1/11 -> Mux2/11  "<Y>"
  Sum/1 -> Bus Creator3/1  "P"
  Bus Selector3/10 -> Mux3/10  "<Xdot>"
  Bus Selector2/10 -> Mux1/10  "<xdot>"
  Reshape1/1 -> Bus Creator3/2  "V"
  Mux2/1 -> Reshape/1
  Bus Selector1/4 -> Mux2/4  "<X>"
  Reshape/1 -> Sum/1
  Bus Selector1/8 -> Mux2/8  "<Y>"
  Bus Selector3/4 -> Mux3/4  "<Xdot>"
  Bus Selector2/2 -> Mux1/2  "<ydot>"
  Mux3/1 -> Reshape1/1
  Mux1/1 -> Reshape2/1
  Bus Selector2/12 -> Mux1/12  "<zdot>"
  Bus Selector2/8 -> Mux1/8  "<ydot>"
  Bus Selector2/9 -> Mux1/9  "<zdot>"
  Bus Creator3/1 -> VehSusp/1  "Veh"
  Bus Selector3/5 -> Mux3/5  "<Ydot>"
  Bus Selector3/11 -> Mux3/11  "<Ydot>"
  Bus Selector1/6 -> Mux2/6  "<Z>"
  Bus Selector2/4 -> Mux1/4  "<xdot>"
  Bus Selector2/11 -> Mux1/11  "<ydot>"
  Bus Selector2/1 -> Mux1/1  "<xdot>"
  Bus Selector1/10 -> Mux2/10  "<X>"
  Bus Selector1/12 -> Mux2/12  "<Z>"

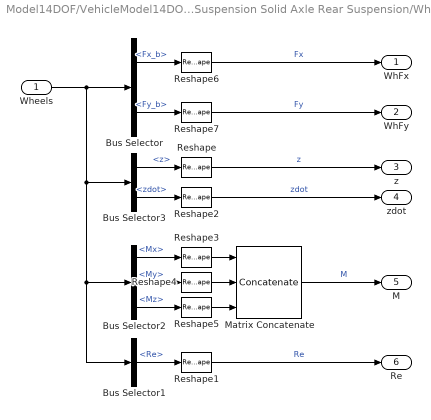
== system Model14DOF/VehicleModel14DOF/MacPherson Front Suspension Solid Axle Rear Suspension/Wheel Adapter ==
  Wheels : Inport
  Bus Selector : BusSelector  OutputSignals=SuspFrame.Fx_b,SuspFrame.Fy_b
  Bus Selector1 : BusSelector  OutputSignals=SuspFrame.Re
  Bus Selector2 : BusSelector  OutputSignals=SuspFrame.Mx,SuspFrame.My,SuspFrame.Mz
  Bus Selector3 : BusSelector  OutputSignals=SuspFrame.z,SuspFrame.zdot
  Matrix Concatenate : Concatenate  NumInputs=3  Mode=Multidimensional array
  Reshape{,1..7} (8 alike) : Reshape  OutputDimensionality=Row vector (2-D)
  WhFx : Outport
  WhFy : Outport  Port=2
  z : Outport  Port=3
  zdot : Outport  Port=4
  M : Outport  Port=5
  Re : Outport  Port=6
  wires:
  Bus Selector/2 -> Reshape7/1  "<Fy_b>"
  Reshape5/1 -> Matrix Concatenate/3
  Reshape4/1 -> Matrix Concatenate/2
  Wheels/1 -> Bus Selector1/1, Bus Selector2/1, Bus Selector3/1, Bus Selector/1
  Reshape/1 -> z/1  "z"
  Bus Selector1/1 -> Reshape1/1  "<Re>"
  Reshape3/1 -> Matrix Concatenate/1
  Bus Selector2/1 -> Reshape3/1  "<Mx>"
  Bus Selector3/1 -> Reshape/1  "<z>"
  Bus Selector3/2 -> Reshape2/1  "<zdot>"
  Bus Selector2/3 -> Reshape5/1  "<Mz>"
  Bus Selector/1 -> Reshape6/1  "<Fx_b>"
  Matrix Concatenate/1 -> M/1  "M"
  Bus Selector2/2 -> Reshape4/1  "<My>"
  Reshape7/1 -> WhFy/1  "Fy"
  Reshape2/1 -> zdot/1  "zdot"
  Reshape1/1 -> Re/1  "Re"
  Reshape6/1 -> WhFx/1  "Fx"

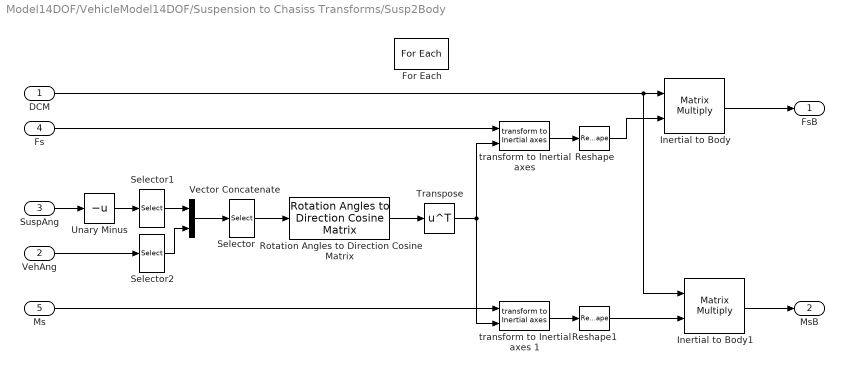
== system Model14DOF/VehicleModel14DOF/Suspension to Chasiss Transforms/Susp2Body ==
  DCM : Inport
  VehAng : Inport  Port=2
  SuspAng : Inport  Port=3
  Fs : Inport  Port=4  Partition=on  PartitionDimension=2  PartitionWidth=1  PartitionOffset=0
  Ms : Inport  Port=5  Partition=on  PartitionDimension=2  PartitionWidth=1  PartitionOffset=0
  For Each : ForEach  DisableCoverage=on
  Inertial to Body : Product  Multiplication=Matrix(*)  InputSameDT=on  SaturateOnIntegerOverflow=on  OutDataTypeStr=Inherit: Same as first input
  Inertial to Body1 : Product  Multiplication=Matrix(*)  InputSameDT=on  SaturateOnIntegerOverflow=on  OutDataTypeStr=Inherit: Same as first input
  Reshape : Reshape
  Reshape1 : Reshape
  Rotation Angles to Direction Cosine Matrix : sharedtransform/Rotation Angles to Direction Cosine Matrix  rotationOrder=ZYX  aMode=2
      settings: SourceProductBaseCode=AE,PW,DR,MT,UV,VE
  Selector : Selector  InputPortWidth=3  IndexOptions=Index vector (dialog)  Indices=[3 2 1]  OutputSizes=1
  Selector1 : Selector  InputPortWidth=3  IndexOptions=Index vector (dialog)  Indices=[1 2]  OutputSizes=1
  Selector2 : Selector  InputPortWidth=3  IndexOptions=Index vector (dialog)  Indices=[3]  OutputSizes=1
  Transpose : Math  Operator=transpose  SignedPower=on  SaturateOnIntegerOverflow=on
  Unary Minus : UnaryMinus
  Vector Concatenate : Concatenate
  "transform to Inertial axes " : shared6dof/6DOF (Euler Angles)/transform to Inertial axes   SystemSampleTime=-1  VariantActivationTime=update diagram  Latency=0  AutoFrameSizeCalculation=off
      settings: SourceProductBaseCode=AE,PW,DR,MT,UV,VE
  transform to Inertial axes 1 : shared6dof/6DOF (Euler Angles)/transform to Inertial axes   SystemSampleTime=-1  VariantActivationTime=update diagram  Latency=0  AutoFrameSizeCalculation=off
      settings: SourceProductBaseCode=AE,PW,DR,MT,UV,VE
  FsB : Outport  ConcatenationDimension=2  VectorParamsAs1DForOutWhenUnconnected=off
  MsB : Outport  Port=2  ConcatenationDimension=2  VectorParamsAs1DForOutWhenUnconnected=off
  wires:
  Reshape/1 -> Inertial to Body/2
  Inertial to Body/1 -> FsB/1
  SuspAng/1 -> Unary Minus/1
  Selector/1 -> Rotation Angles to Direction Cosine Matrix/1
  Fs/1 -> "transform to Inertial axes "/1
  Transpose/1 -> transform to Inertial axes 1/2, "transform to Inertial axes "/2
  Rotation Angles to Direction Cosine Matrix/1 -> Transpose/1
  "transform to Inertial axes "/1 -> Reshape/1
  transform to Inertial axes 1/1 -> Reshape1/1
  Inertial to Body1/1 -> MsB/1
  Reshape1/1 -> Inertial to Body1/2
  DCM/1 -> Inertial to Body1/1, Inertial to Body/1
  Ms/1 -> transform to Inertial axes 1/1
  VehAng/1 -> Selector2/1
  Unary Minus/1 -> Selector1/1
  Selector1/1 -> Vector Concatenate/1
  Vector Concatenate/1 -> Selector/1
  Selector2/1 -> Vector Concatenate/2

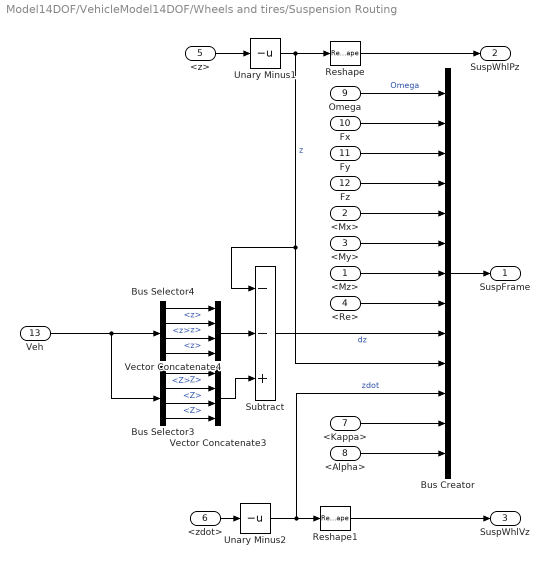
== system Model14DOF/VehicleModel14DOF/Wheels and tires/Suspension Routing ==
  <Mz> : Inport
  <Mx> : Inport  Port=2
  <My> : Inport  Port=3
  <Re> : Inport  Port=4
  <z> : Inport  Port=5
  <zdot> : Inport  Port=6
  <Kappa> : Inport  Port=7
  <Alpha> : Inport  Port=8
  Omega : Inport  Port=9
  Fx : Inport  Port=10
  Fy : Inport  Port=11
  Fz : Inport  Port=12
  Veh : Inport  Port=13
  Bus Creator : BusCreator  Inputs=13
  Bus Selector3 : BusSelector  OutputSignals=InertFrm.FrntAxl.Lft.Disp.Z,InertFrm.FrntAxl.Rght.Disp.Z,InertFrm.RearAxl.Lft.Disp.Z,InertFrm.RearAxl.Rght.Disp.Z
  Bus Selector4 : BusSelector  OutputSignals=BdyFrm.FrntAxl.Lft.Disp.z,BdyFrm.FrntAxl.Rght.Disp.z,BdyFrm.RearAxl.Lft.Disp.z,BdyFrm.RearAxl.Rght.Disp.z
  Reshape : Reshape  OutputDimensionality=Row vector (2-D)
  Reshape1 : Reshape  OutputDimensionality=Row vector (2-D)
  Subtract : Sum  Inputs=--+
  Unary Minus1 : UnaryMinus
  Unary Minus2 : UnaryMinus
  Vector Concatenate3 : Concatenate  NumInputs=4
  Vector Concatenate4 : Concatenate  NumInputs=4
  SuspFrame : Outport  VectorParamsAs1DForOutWhenUnconnected=off
  SuspWhlPz : Outport  Port=2  VectorParamsAs1DForOutWhenUnconnected=off
  SuspWhlVz : Outport  Port=3  VectorParamsAs1DForOutWhenUnconnected=off
  wires:
  <Re>/1 -> Bus Creator/8
  Unary Minus1/1 -> Bus Creator/10, Subtract/1, Reshape/1  "z"
  Fz/1 -> Bus Creator/4
  <zdot>/1 -> Unary Minus2/1
  <Mz>/1 -> Bus Creator/7
  Unary Minus2/1 -> Bus Creator/11, Reshape1/1  "zdot"
  <z>/1 -> Unary Minus1/1
  Bus Creator/1 -> SuspFrame/1
  Fy/1 -> Bus Creator/3
  Omega/1 -> Bus Creator/1  "Omega"
  Fx/1 -> Bus Creator/2
  Reshape1/1 -> SuspWhlVz/1
  <Kappa>/1 -> Bus Creator/12
  Reshape/1 -> SuspWhlPz/1
  <Mx>/1 -> Bus Creator/5
  <My>/1 -> Bus Creator/6
  <Alpha>/1 -> Bus Creator/13
  Veh/1 -> Bus Selector3/1, Bus Selector4/1
  Bus Selector3/4 -> Vector Concatenate3/4  "<Z>"
  Subtract/1 -> Bus Creator/9  "dz"
  Bus Selector4/1 -> Vector Concatenate4/1  "<z>"
  Bus Selector3/1 -> Vector Concatenate3/1  "<Z>"
  Vector Concatenate3/1 -> Subtract/3
  Vector Concatenate4/1 -> Subtract/2
  Bus Selector4/2 -> Vector Concatenate4/2  "<z>"
  Bus Selector3/3 -> Vector Concatenate3/3  "<Z>"
  Bus Selector3/2 -> Vector Concatenate3/2  "<Z>"
  Bus Selector4/4 -> Vector Concatenate4/4  "<z>"
  Bus Selector4/3 -> Vector Concatenate4/3  "<z>"

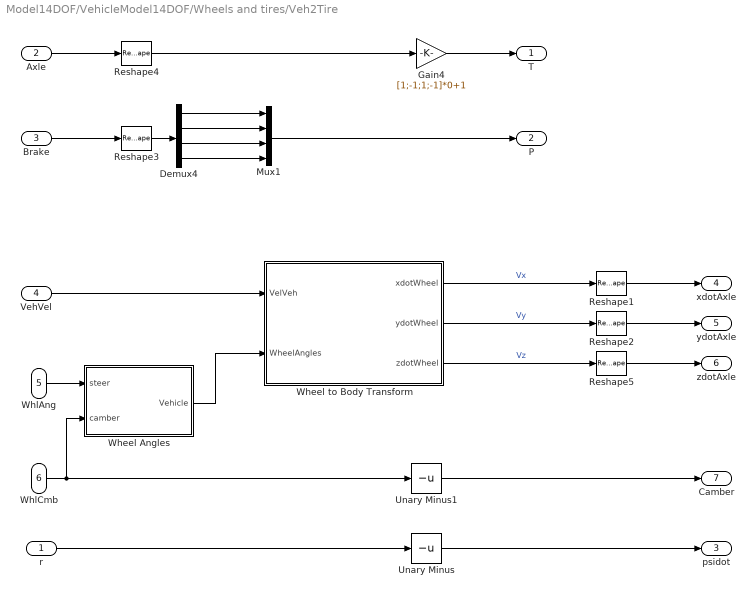
== system Model14DOF/VehicleModel14DOF/Wheels and tires/Veh2Tire ==
  r : Inport
  Axle : Inport  Port=2
  Brake : Inport  Port=3
  VehVel : Inport  Port=4
  WhlAng : Inport  Port=5
  WhlCmb : Inport  Port=6
  Demux4 : Demux
  Gain4 : Gain  Gain=[1;-1;1;-1]*0+1
  Mux1 : Mux
  Reshape{1..5} (5 alike) : Reshape
  Unary Minus : UnaryMinus
  Unary Minus1 : UnaryMinus
  Wheel Angles : Subsystem
  Wheel to Body Transform : Subsystem
  T : Outport  Unit=N*m  VectorParamsAs1DForOutWhenUnconnected=off
  P : Outport  Port=2  Unit=Pa  VectorParamsAs1DForOutWhenUnconnected=off
  psidot : Outport  Port=3  Unit=rad/s  VectorParamsAs1DForOutWhenUnconnected=off
  xdotAxle : Outport  Port=4  Unit=m/s  VectorParamsAs1DForOutWhenUnconnected=off
  ydotAxle : Outport  Port=5  Unit=m/s  VectorParamsAs1DForOutWhenUnconnected=off
  zdotAxle : Outport  Port=6  Unit=m/s  VectorParamsAs1DForOutWhenUnconnected=off
  Camber : Outport  Port=7  Unit=rad  VectorParamsAs1DForOutWhenUnconnected=off
  wires:
  Demux4/1 -> Mux1/1
  Brake/1 -> Reshape3/1
  Demux4/4 -> Mux1/4
  Axle/1 -> Reshape4/1
  Wheel to Body Transform/1(xdotWheel) -> Reshape1/1  "Vx"
  Demux4/2 -> Mux1/2
  Wheel to Body Transform/2(ydotWheel) -> Reshape2/1  "Vy"
  WhlAng/1 -> Wheel Angles/1(steer)
  Mux1/1 -> P/1
  r/1 -> Unary Minus/1
  Demux4/3 -> Mux1/3
  Reshape3/1 -> Demux4/1
  Gain4/1 -> T/1
  Reshape4/1 -> Gain4/1
  VehVel/1 -> Wheel to Body Transform/1(VelVeh)
  Wheel to Body Transform/3(zdotWheel) -> Reshape5/1  "Vz"
  WhlCmb/1 -> Unary Minus1/1, Wheel Angles/2(camber)
  Unary Minus/1 -> psidot/1
  Wheel Angles/1(Vehicle) -> Wheel to Body Transform/2(WheelAngles)
  Reshape1/1 -> xdotAxle/1
  Reshape2/1 -> ydotAxle/1
  Reshape5/1 -> zdotAxle/1
  Unary Minus1/1 -> Camber/1

== system Model14DOF/VehicleModel14DOF/Wheels and tires/Wheel Angles ==
  Front : Inport
  Camber : Inport  Port=2
  Constant : Constant  Value=zeros(4,1)
  Reshape : Reshape  OutputDimensionality=Row vector (2-D)
  Reshape1 : Reshape  OutputDimensionality=Row vector (2-D)
  Reshape2 : Reshape  OutputDimensionality=Row vector (2-D)
  Vector Concatenate3 : Concatenate  NumInputs=3  Mode=Multidimensional array
  Vehicle : Outport  VectorParamsAs1DForOutWhenUnconnected=off
  wires:
  Reshape/1 -> Vector Concatenate3/3
  Reshape2/1 -> Vector Concatenate3/2
  Vector Concatenate3/1 -> Vehicle/1
  Reshape1/1 -> Vector Concatenate3/1
  Front/1 -> Reshape/1
  Camber/1 -> Reshape1/1
  Constant/1 -> Reshape2/1
